simulink model "lab3_3"  (R2023b)
settings: Solver=FixedStepAuto  StartTime=0.0  StopTime=100  FixedStep=1  RelTol=1e-3
values from neighbouring files (symbols this model uses):
  delta = deltas(i)    [lab3_56.m]
settings Model: Creator=user  LastModifiedBy=Admin

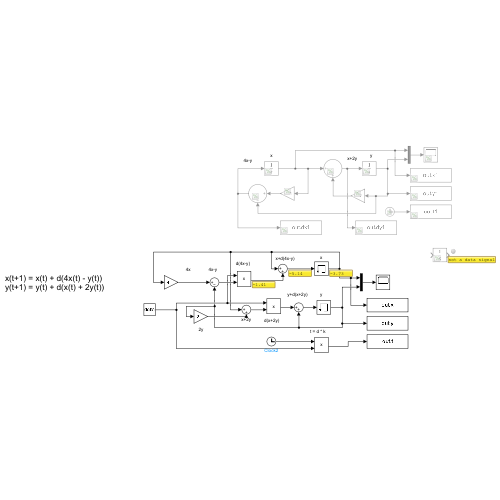
[thumbnail: Simulink's stored preview of the top-level diagram]
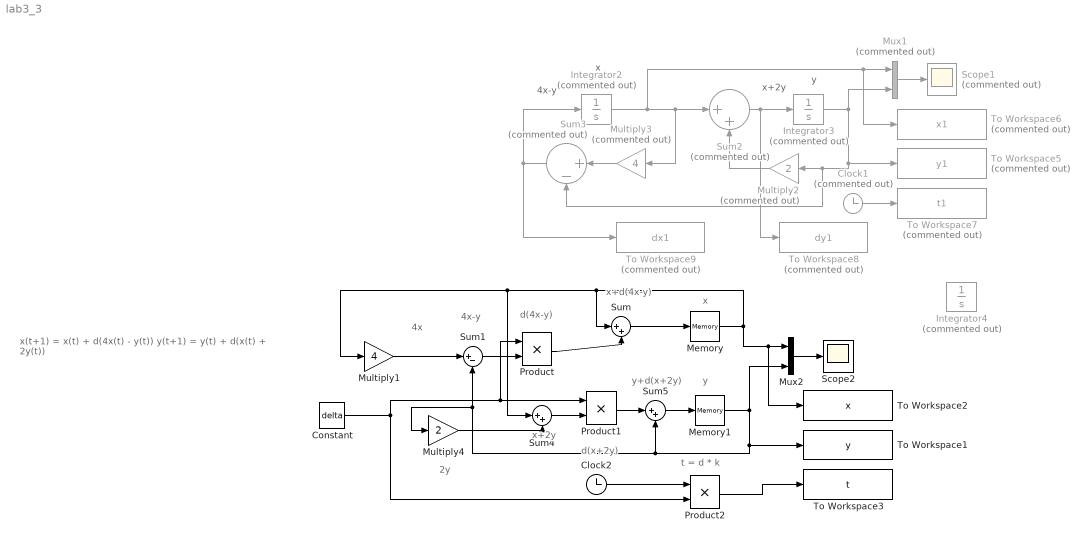
== system lab3_3 ==
  note: t = d * k
  note: y+d(x+2y)
  note: d(x+2y)
  note: x+2y
  note: 2y
  note: x+d(4x-y)
  note: d(4x-y)
  note: 4x-y
  note: 4x
  note: y
  note: 4x-y
  note: x
  note: x+2y
  note: x(t+1) = x(t) + d(4x(t) - y(t))
      | y(t+1) = y(t) + d(x(t) + 2y(t))
  note: x
  note: y
  Clock1 : Clock  Commented=on
  Clock2 : Clock
  Constant : Constant  Value=delta
  Integrator2 : Integrator  Commented=on  InitialCondition=-1
  Integrator3 : Integrator  Commented=on
  Integrator4 : Integrator  Commented=on  InitialCondition=-1
  Memory : Memory  InitialCondition=-1
  Memory1 : Memory
  Multiply1 : Gain  Gain=4
  Multiply2 : Gain  Commented=on  Gain=2
  Multiply3 : Gain  Commented=on  Gain=4
  Multiply4 : Gain  Gain=2
  Mux1 : Mux  Commented=on  Inputs=2
  Mux2 : Mux  Inputs=2
  Product : Product
  Product1 : Product
  Product2 : Product
  Scope1 : Scope  Commented=on
  Scope2 : Scope
  Sum : Sum  Inputs=|++
  Sum1 : Sum  Inputs=|+-
  Sum2 : Sum  Commented=on  Inputs=|++
  Sum3 : Sum  Commented=on  Inputs=|+-
  Sum4 : Sum  Inputs=|++
  Sum5 : Sum  Inputs=|++
  To Workspace1 : ToWorkspace  VariableName=y  SampleTime=-1
  To Workspace2 : ToWorkspace  VariableName=x  SampleTime=-1
  To Workspace3 : ToWorkspace  VariableName=t  SampleTime=-1
  To Workspace5 : ToWorkspace  Commented=on  VariableName=y1  SampleTime=-1
  To Workspace6 : ToWorkspace  Commented=on  VariableName=x1  SampleTime=-1
  To Workspace7 : ToWorkspace  Commented=on  VariableName=t1  SampleTime=-1
  To Workspace8 : ToWorkspace  Commented=on  VariableName=dy1  SampleTime=-1
  To Workspace9 : ToWorkspace  Commented=on  VariableName=dx1  SampleTime=-1
  wires:
  Integrator3/1 -> To Workspace5/1, Sum3/2, Multiply2/1, Mux1/2
  Integrator2/1 -> Multiply3/1, Sum2/1, To Workspace6/1, Mux1/1
  Sum2/1 -> To Workspace8/1, Integrator3/1
  Mux1/1 -> Scope1/1
  Multiply3/1 -> Sum3/1
  Sum3/1 -> To Workspace9/1, Integrator2/1
  Clock1/1 -> To Workspace7/1
  Multiply2/1 -> Sum2/2
  Memory/1 -> To Workspace2/1, Mux2/1, Sum4/1, Multiply1/1, Sum/1
  Constant/1 -> Product1/1, Product/1, Product2/2
  Memory1/1 -> Mux2/2, To Workspace1/1, Multiply4/1, Sum1/2, Sum5/2
  Sum1/1 -> Product/2
  Multiply1/1 -> Sum1/1
  Product/1 -> Sum/2
  Sum/1 -> Memory/1
  Sum4/1 -> Product1/2
  Sum5/1 -> Memory1/1
  Product1/1 -> Sum5/1
  Multiply4/1 -> Sum4/2
  Mux2/1 -> Scope2/1
  Clock2/1 -> Product2/1
  Product2/1 -> To Workspace3/1
